simulink model "o1_ar_filter_sim"  (R2020b)
settings: Solver=FixedStepDiscrete  StartTime=0.0  StopTime=stopTime  RelTol=1e-3
InitFcn:
  | initCallback
StopFcn:
  | stopCallback
values from neighbouring files (symbols this model uses):
  buf_random_in = rand(1,1)    [modelparameters.m]
  c1_a_random_in = rand(1,1)    [modelparameters.m]
  c1_r_random_in = rand(1,1)    [modelparameters.m]
  c2_a_random_in = rand(1,1)    [modelparameters.m]
  c2_r_random_in = rand(1,1)    [modelparameters.m]
undefined symbols (not defined in the file or in its folder): mp
settings Model: Creator=Ross  LastModifiedBy=conno
settings DataIOCC: ReturnWorkspaceOutputs=off
settings OptimizationCC: BlockReduction=off  ConditionallyExecuteInputs=off  DefaultParameterBehavior=Inlined
settings DebuggingCC: ReadBeforeWriteMsg=DisableAll  WriteAfterWriteMsg=DisableAll  WriteAfterReadMsg=DisableAll  AlgebraicLoopMsg=error  MultiTaskDSMMsg=none  SingleTaskRateTransMsg=error  PregeneratedLibrarySubsystemCodeDiagnostic=none  ArithmeticOperatorsInVariantConditions=warning
settings HardwareCC: ProdBitPerPointer=32  ProdBitPerSizeT=32  ProdBitPerPtrDiffT=32  ProdLargestAtomicFloat=None  ProdIntDivRoundTo=Undefined  ProdEndianess=Unspecified  ProdWordSize=32  ProdHWDeviceType=ASIC/FPGA->ASIC/FPGA  TargetBitPerPointer=64  TargetBitPerSizeT=64  TargetBitPerPtrDiffT=64  TargetLongLongMode=on  TargetIntDivRoundTo=Zero  TargetEndianess=LittleEndian  TargetWordSize=64  TargetHWDeviceType=Custom Processor->MATLAB Host Computer  ProdEqTarget=off
settings ModelReferenceCC: UpdateModelReferenceTargets=IfOutOfDate
settings SFSimCC: SFSimEcho=off  SimUseLocalCustomCode=off  CustomCodeUndefinedFunction=UseInterfaceOnly
settings RTWCC: RTWUseLocalCustomCode=off

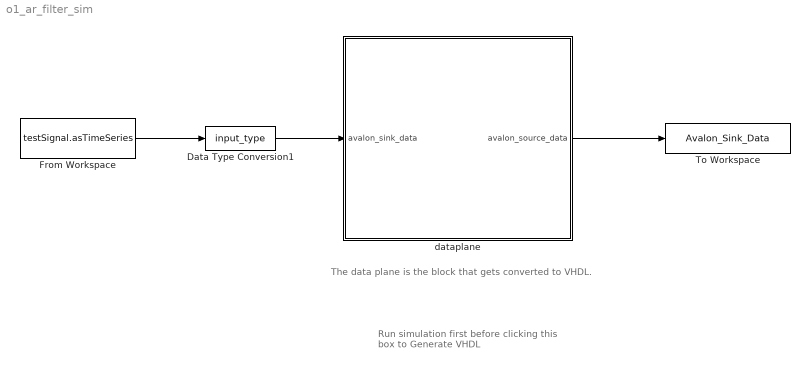
== system o1_ar_filter_sim ==
  note: The data plane is the block that gets converted to VHDL.
  note: Run simulation first
      | before clicking this box to
      | Generate VHDL
  Data Type Conversion1 : DataTypeConversion  OutDataTypeStr=input_type  RndMeth=Nearest
  From Workspace : FromWorkspace  VariableName=testSignal.asTimeSeries  SampleTime=mp.Ts
  To Workspace : ToWorkspace  VariableName=Avalon_Sink_Data  SampleTime=-1
  dataplane : Subsystem  TreatAsAtomicUnit=on
  wires:
  dataplane/1(avalon_source_data) -> To Workspace/1
  Data Type Conversion1/1 -> dataplane/1(avalon_sink_data)
  From Workspace/1 -> Data Type Conversion1/1

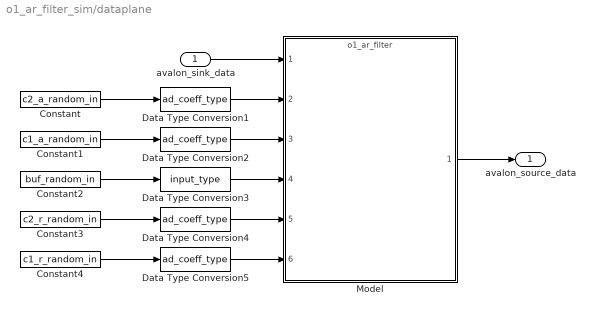
== system o1_ar_filter_sim/dataplane ==
  avalon_sink_data : Inport
  Constant : Constant  Value=c2_a_random_in  SampleTime=-1
  Constant1 : Constant  Value=c1_a_random_in  SampleTime=-1
  Constant2 : Constant  Value=buf_random_in  SampleTime=-1
  Constant3 : Constant  Value=c2_r_random_in  SampleTime=-1
  Constant4 : Constant  Value=c1_r_random_in  SampleTime=-1
  Data Type Conversion{1..2,4..5} (4 alike) : DataTypeConversion  OutDataTypeStr=ad_coeff_type  RndMeth=Nearest
  Data Type Conversion3 : DataTypeConversion  OutDataTypeStr=input_type  RndMeth=Nearest
  Model : ModelReference  ModelNameDialog=o1_ar_filter.slx  SimulationMode=Normal  ModelReferenceVersion=1.152
  avalon_source_data : Outport  VectorParamsAs1DForOutWhenUnconnected=off
  wires:
  avalon_sink_data/1 -> Model/1
  Model/1 -> avalon_source_data/1
  Data Type Conversion1/1 -> Model/2
  Constant/1 -> Data Type Conversion1/1
  Data Type Conversion3/1 -> Model/4
  Constant2/1 -> Data Type Conversion3/1
  Data Type Conversion2/1 -> Model/3
  Constant1/1 -> Data Type Conversion2/1
  Data Type Conversion5/1 -> Model/6
  Data Type Conversion4/1 -> Model/5
  Constant4/1 -> Data Type Conversion5/1
  Constant3/1 -> Data Type Conversion4/1
